simulink model "DSB"  (R2019b)
settings: Solver=VariableStepAuto  StartTime=0.0  StopTime=10  RelTol=1e-3
libraries: commanapbnd3 x2, eeGeneralControl x1
settings Model: Creator=thuma  LastModifiedBy=thuma

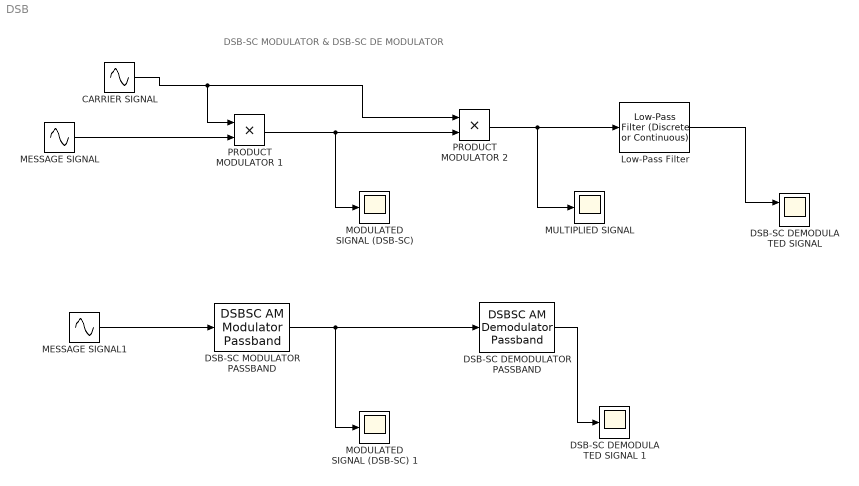
== system DSB ==
  note: DSB-SC MODULATOR & DSB-SC DE MODULATOR
  " DSB-SC DEMODULATOR PASSBAND" : commanapbnd3/DSBSC AM Demodulator Passband  Fc=20  Ph=0  method=Butterworth  n=4  cf=1  Rp=0.1  Rs=50
      settings: SourceProductName=Communications Toolbox  SourceProductBaseCode=CM
  " DSB-SC MODULATOR PASSBAND" : commanapbnd3/DSBSC AM Modulator Passband  Fc=20  Ph=0
      settings: SourceProductName=Communications Toolbox  SourceProductBaseCode=CM
  " DSB-SC DEMODULATED SIGNAL 1" : Scope
  " DSB-SC DEMODULATED SIGNAL " : Scope  NumInputPorts=2
  " Low-Pass Filter " : eeGeneralControl/Low-Pass Filter (Discrete or Continuous)  K=1  T=1  B=1  A=-1  Ts=0
      settings: SourceProductName=Simscape Electrical
  CARRIER SIGNAL : Sin  Frequency=100  SampleTime=0
  MESSAGE SIGNAL : Sin  SampleTime=0
  MESSAGE SIGNAL1 : Sin  Frequency=2*pi*1  SampleTime=0.001
  MODULATED SIGNAL (DSB-SC) : Scope
  MODULATED SIGNAL (DSB-SC) 1 : Scope
  MULTIPLIED SIGNAL : Scope
  PRODUCT MODULATOR 1 : Product
  PRODUCT MODULATOR 2 : Product
  wires:
  PRODUCT MODULATOR 1/1 -> PRODUCT MODULATOR 2/2, MODULATED SIGNAL (DSB-SC)/1
  PRODUCT MODULATOR 2/1 -> " Low-Pass Filter "/1, MULTIPLIED SIGNAL/1
  MESSAGE SIGNAL/1 -> PRODUCT MODULATOR 1/2
  CARRIER SIGNAL/1 -> PRODUCT MODULATOR 2/1, PRODUCT MODULATOR 1/1
  " Low-Pass Filter "/1 -> " DSB-SC DEMODULATED SIGNAL "/1
  MESSAGE SIGNAL1/1 -> " DSB-SC MODULATOR PASSBAND"/1
  " DSB-SC MODULATOR PASSBAND"/1 -> " DSB-SC DEMODULATOR PASSBAND"/1, MODULATED SIGNAL (DSB-SC) 1/1
  " DSB-SC DEMODULATOR PASSBAND"/1 -> " DSB-SC DEMODULATED SIGNAL 1"/1
